simulink model "code_gen_man_bin"  (Simulink 7.5)
settings: Solver=FixedStepDiscrete  SolverMode=SingleTasking  StartTime=0.0  StopTime=10.0  FixedStep=0.01  RelTol=1e-3
InitFcn:
  | boat_constants
values from neighbouring files (symbols this model uses):
  figure8_waypoints = int32([ ... (first row only)    [boat_constants.m]
  InitialPoint = 0    [boat_constants.m]    (also in l2plus.m)
  IPStar = 0    [boat_constants.m]    (also in l2plus.m)
  ISA_g = 9.815    [boat_constants.m]
  MaxDwnPthStar = 1    [boat_constants.m]    (also in l2plus.m)
  OC2max = 49999    [boat_constants.m]    (also in simulation_constants.m)
  sampling_waypoints = int32([ ... (first row only)    [boat_constants.m]
  switchDistance = 4    [boat_constants.m]    (also in l2plus.m)
  T_step = 0.01    [boat_constants.m]    (also in common.m)
  tanIntercept = tan( 45*pi/180 )    [boat_constants.m]    (also in l2plus.m)
  test_waypoints = int32([ ... (first row only)    [boat_constants.m]
  TStar = single(4.5)    [boat_constants.m]    (also in l2plus.m = single(2))
  Turn2Track = 0    [boat_constants.m]    (also in l2plus.m)
  wheelbase = 3.27    [boat_constants.m]
undefined symbols (not defined in the file or in its folder): clearGpsData, clearSensorData, cpInitCommunications, DataEEInitAndClear, DataEEWrite, DiscIntNeverNeededParam, ecan1_buffered_transmit_matlab, ecan1_error_status_matlab, ecan1_init, GetAirData, getGpsData, getRevoData, getSensorData, GetThrottleData, GetWaterData, GetWindData, Init_onlyOnce, Init_Reset, initCalibrationRange, initGps, processNewCommData, processNewGpsData, processNewRevoData, setHilMode, u1, u2, uart1EnqueueStateData, uart2EnqueueActuatorData, y1
libraries: simulink x80, dsPICdrivers x50, uSimLib x4, simulink_need_slupdate x4
(part 3 of 6)

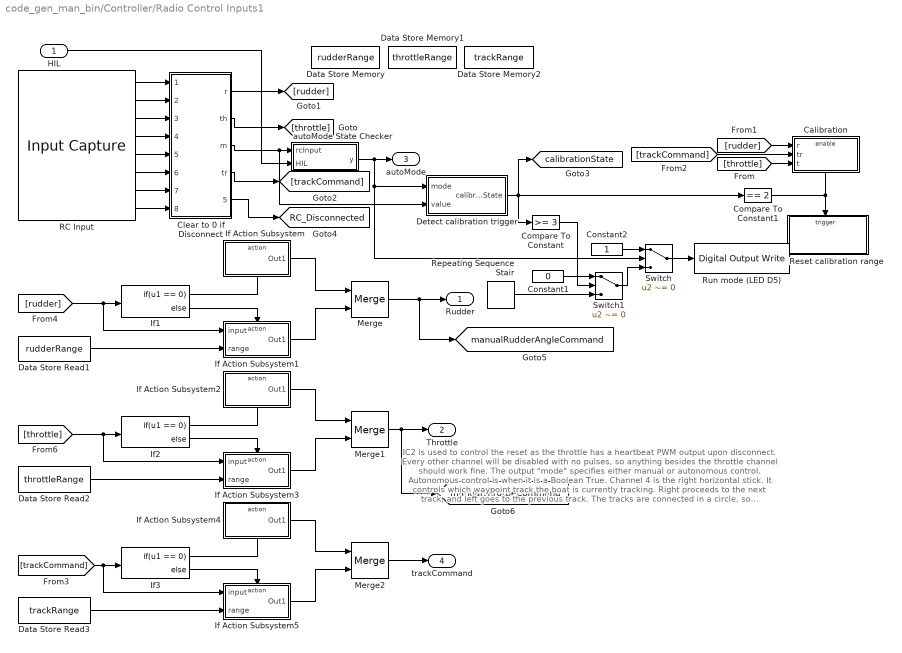
== system code_gen_man_bin/Controller/Radio Control Inputs1 ==
  note: IC2 is used to control the reset as the throttle has a heartbeat PWM output upon disconnect.
      | Every other channel will be disabled with no pulses, so anything besides the throttle channel
      | should work fine.
      |
      | The output "mode" specifies either manual or autonomous control. Autonomous control is when
      | it is a Boolean True.
      |
      | Channel 4 is the right horizontal stick. It controls which waypoint track the boat is currently tracking.
      | Right proceeds to the next track, and left goes to the previous track. The tracks are connected in a
      | circle, so next/prevTrack will eventually wrap around.
      |
      | All controls for the vehicle are controlled when AutoMode is True. When the vehicle is in
      | AutoMode, then its calibration features are engaged. Moving all control channels besides channel
      | 5 (which is reserved for switching AutoMode) will calibrate the controller to the proper values.
      |
      | As the vehicle enters reset automatically on startup, the proper way to calibrate is to startup the vehicle.
      | Move all the control sticks (excl channel 5 again) and then switch into RC mode. Even if the vessel stays
      | in reset mode, it will still be controllable via the RC transmitter.
      |
      | The output for rudder, throttle, and trackCommand are all in the range -1..1000. -1 means disconnected,
      | while 0 is a low RC signal and 1000 is a high. These ranges also have deadbands: 4% at the low-end or
      | 8% around the center. This helps to keep the actuator dead if the user desires it.
  HIL : Inport
  Calibration : Subsystem  TreatAsAtomicUnit=on
  Clear to 0 if Disconnect : Subsystem
  Compare To Constant : simulink/Logic and Bit Operations/Compare To Constant  SystemSampleTime=-1  relop=>=  const=3  LogicOutDataTypeMode=boolean
  Compare To Constant1 : simulink/Logic and Bit Operations/Compare To Constant  SystemSampleTime=-1  relop===  const=2  LogicOutDataTypeMode=boolean
  Constant1 : Constant  Value=0  OutDataTypeMode=boolean  OutDataType=fixdt(1, 16)  OutScaling=2^0  OutDataTypeStr=boolean
  Constant2 : Constant  OutDataTypeMode=boolean  OutDataType=fixdt(1, 16)  OutScaling=2^0  OutDataTypeStr=boolean
  Data Store Memory : DataStoreMemory  DataStoreName=rudderRange  ReadBeforeWriteMsg=warning  WriteAfterWriteMsg=warning  WriteAfterReadMsg=warning  InitialValue=[0 0]  DataType=int16  OutDataType=fixdt(1, 16)  OutScaling=2^0  OutDataTypeStr=int16
      settings: RTWStateStorageClass=ExportedGlobal
  Data Store Memory1 : DataStoreMemory  DataStoreName=throttleRange  ReadBeforeWriteMsg=warning  WriteAfterWriteMsg=warning  WriteAfterReadMsg=warning  InitialValue=[8000 8000]  DataType=int16  OutDataType=fixdt(1, 16)  OutScaling=2^0  OutDataTypeStr=int16
      settings: RTWStateStorageClass=ExportedGlobal
  Data Store Memory2 : DataStoreMemory  DataStoreName=trackRange  ReadBeforeWriteMsg=warning  WriteAfterWriteMsg=warning  WriteAfterReadMsg=warning  InitialValue=[8000 8000]  DataType=int16  OutDataType=fixdt(1, 16)  OutScaling=2^0  OutDataTypeStr=int16
      settings: RTWStateStorageClass=ExportedGlobal
  Data Store Read1 : DataStoreRead  DataStoreName=rudderRange  SampleTime=T_step
  Data Store Read2 : DataStoreRead  DataStoreName=throttleRange  SampleTime=T_step
  Data Store Read3 : DataStoreRead  DataStoreName=trackRange  SampleTime=T_step
  Detect calibration trigger : Subsystem
  If Action Subsystem : Subsystem  TreatAsAtomicUnit=on
  If Action Subsystem1 : Subsystem  TreatAsAtomicUnit=on
  If Action Subsystem2 : Subsystem  TreatAsAtomicUnit=on
  If Action Subsystem3 : Subsystem  TreatAsAtomicUnit=on
  If Action Subsystem4 : Subsystem  TreatAsAtomicUnit=on
  If Action Subsystem5 : Subsystem  TreatAsAtomicUnit=on
  If1 : If  IfExpression=u1 == 0
  If2 : If  IfExpression=u1 == 0
  If3 : If  IfExpression=u1 == 0
  Merge : Merge
  Merge1 : Merge
  Merge2 : Merge
  RC Input : dsPICdrivers/Peripheral I//O/Input Capture  Tag=dsPIC_PWM_IC  Priority=5  IntPriority=7  Channel=[2 3 4 8]  Channel_UP_Down_Periode="[1  1  1  1]"  MaxChannel="[0.0025      0.0025      0.0025      0.0025]"  SafeMarge="[1  1  1  1]"  MaxName=' IC2max , IC3max , IC4max , IC8max '  Precision="[13.6094      13.6094      13.6094      13.6094]"  Timer="[2  2  2  2]"  ChangeDetected="[2  2  2  2]"  ChangeDetectedPortRef=3  SampleTime=.01  Status=OK
  Repeating Sequence Stair : simulink/Sources/Repeating Sequence Stair  SystemSampleTime=-1  OutValues=[1 1 1 1 1 1 1 1 1 1 0 0 0 0 0 0 0 0 0 0]  tsamp=.01  OutMin=[]  OutMax=[]  OutDataTypeStr=fixdt('boolean')  OutputDataTypeScalingMode=Specify via dialog  OutDataType=fixdt('boolean')  ConRadixGroup=Best Precision: Vector-wise  OutScaling=[]
  Reset calibration range : Subsystem  TreatAsAtomicUnit=on
  Run mode (LED D5) : dsPICdrivers/Digital I//O/Digital Output Write  Tag=dsPIC_Digital_Output  Priority=5  PORT=A  Pin=[2]  Simultaneous=off  OrderingInOutPopup=None
  Switch : Switch  Criteria=u2 ~= 0  OutDataType=fixdt(1, 16)  OutScaling=2^0
  Switch1 : Switch  Criteria=u2 ~= 0  OutDataType=fixdt(1, 16)  OutScaling=2^0
  autoMode State Checker : Stateflow chart  TreatAsAtomicUnit=on
  Rudder : Outport
  Throttle : Outport  Port=2
  autoMode : Outport  Port=3
  trackCommand : Outport  Port=4
  tag scope: RC_Disconnected=global, calibrationState=global, manualRudderAngleCommand=global, manualThrottleCommand=global
  wires:
  Clear to 0 if Disconnect/3(m) -> Detect calibration trigger/2(value), autoMode State Checker/1(rcInput)
  Clear to 0 if Disconnect/1(r) -> [rudder]
  Clear to 0 if Disconnect/2(th) -> [throttle]
  Clear to 0 if Disconnect/4(tr) -> [trackCommand]
  [rudder] -> If Action Subsystem1/1(input), If1/1
  Data Store Read2/1 -> If Action Subsystem3/2(range)
  If1/1 -> If Action Subsystem/Action
  If1/2 -> If Action Subsystem1/Action
  If Action Subsystem1/1(Out1) -> Merge/2
  If Action Subsystem/1(Out1) -> Merge/1
  Data Store Read1/1 -> If Action Subsystem1/2(range)
  [throttle] -> If2/1, If Action Subsystem3/1(input)
  Merge1/1 -> Throttle/1, [manualThrottleCommand]
  If2/1 -> If Action Subsystem2/Action
  If2/2 -> If Action Subsystem3/Action
  If Action Subsystem3/1(Out1) -> Merge1/2
  If Action Subsystem2/1(Out1) -> Merge1/1
  [trackCommand] -> If3/1, If Action Subsystem5/1(input)
  Merge2/1 -> trackCommand/1
  If3/1 -> If Action Subsystem4/Action
  If3/2 -> If Action Subsystem5/Action
  If Action Subsystem5/1(Out1) -> Merge2/2
  If Action Subsystem4/1(Out1) -> Merge2/1
  Data Store Read3/1 -> If Action Subsystem5/2(range)
  autoMode State Checker/1(y) -> autoMode/1, Detect calibration trigger/1(mode), Switch/2
  Detect calibration trigger/1(calibrateState) -> Compare To Constant/1, Compare To Constant1/1, [calibrationState]
  [rudder] -> Calibration/1(r)
  [trackCommand] -> Calibration/2(tr)
  [throttle] -> Calibration/3(t)
  HIL/1 -> autoMode State Checker/2(HIL)
  Compare To Constant1/1 -> Reset calibration range/Trigger, Calibration/Enable
  Switch/1 -> Run mode (LED D5)/1
  Constant2/1 -> Switch/1
  Switch1/1 -> Switch/3
  Repeating Sequence Stair/1 -> Switch1/3
  Compare To Constant/1 -> Switch1/2
  Constant1/1 -> Switch1/1
  RC Input/1 -> Clear to 0 if Disconnect/1(rudder_up)
  RC Input/2 -> Clear to 0 if Disconnect/2(rudder_fall)
  RC Input/3 -> Clear to 0 if Disconnect/3(throttle_up)
  RC Input/4 -> Clear to 0 if Disconnect/4(throttle_fall)
  RC Input/5 -> Clear to 0 if Disconnect/5(mode_up)
  RC Input/6 -> Clear to 0 if Disconnect/6(mode_fall)
  RC Input/7 -> Clear to 0 if Disconnect/7(track_up)
  RC Input/8 -> Clear to 0 if Disconnect/8(track_fall)
  Clear to 0 if Disconnect/5(discon) -> [RC_Disconnected]
  Merge/1 -> Rudder/1, [manualRudderAngleCommand]

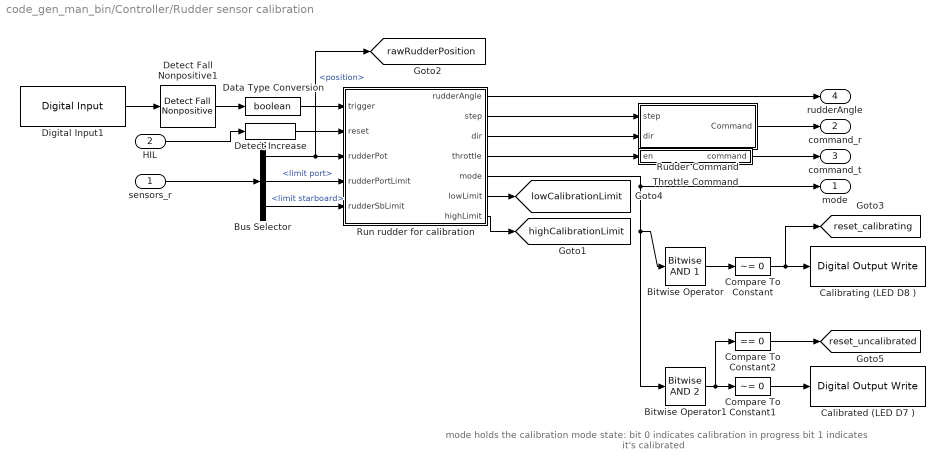
== system code_gen_man_bin/Controller/Rudder sensor calibration ==
  note: mode holds the calibration mode state:
      | bit 0 indicates calibration in progress
      | bit 1 indicates it's calibrated
  sensors_r : Inport
  HIL : Inport  Port=2
  Bitwise Operator : simulink/Logic and Bit Operations/Bitwise Operator  logicop=AND  UseBitMask=on  BitMask=1  BitMaskRealWorld=Stored Integer
  Bitwise Operator1 : simulink/Logic and Bit Operations/Bitwise Operator  logicop=AND  UseBitMask=on  BitMask=2  BitMaskRealWorld=Stored Integer
  Bus Selector : BusSelector  OutputSignals=position,limit port,limit starboard
  Calibrated (LED D7 ) : dsPICdrivers/Digital I//O/Digital Output Write  Tag=dsPIC_Digital_Output  Priority=5  PORT=A  Pin=[4]  Simultaneous=off  OrderingInOutPopup=None
  Calibrating (LED D8 ) : dsPICdrivers/Digital I//O/Digital Output Write  Tag=dsPIC_Digital_Output  Priority=5  PORT=A  Pin=[5]  Simultaneous=off  OrderingInOutPopup=None
  Compare To Constant : simulink/Logic and Bit Operations/Compare To Constant  SystemSampleTime=-1  relop=~=  const=0  LogicOutDataTypeMode=boolean
  Compare To Constant1 : simulink/Logic and Bit Operations/Compare To Constant  SystemSampleTime=-1  relop=~=  const=0  LogicOutDataTypeMode=boolean
  Compare To Constant2 : simulink/Logic and Bit Operations/Compare To Constant  SystemSampleTime=-1  relop===  const=0  LogicOutDataTypeMode=boolean
  Data Type Conversion : DataTypeConversion  OutDataTypeMode=boolean  OutDataType=fixdt(1, 16)  OutScaling=2^0  OutDataTypeStr=boolean
  Detect Increase : simulink/Logic and Bit Operations/Detect Increase  SystemSampleTime=-1  vinit=0.0
  Detect Fall Nonpositive1 : simulink/Logic and Bit Operations/Detect Fall Nonpositive  SystemSampleTime=-1  vinit=1
  Digital Input1 : dsPICdrivers/Digital I//O/Digital Input  Tag=dsPIC_Digital_Input  PORT=D  Pin=[7]  SampleTime=T_step  OrderingInOutPopup=None
  Rudder Command : Subsystem
  Run rudder for calibration : Stateflow chart  TreatAsAtomicUnit=on
  Throttle Command : Subsystem
  mode : Outport
  command_r : Outport  Port=2
  command_t : Outport  Port=3
  rudderAngle : Outport  Port=4
  tag scope: highCalibrationLimit=global, lowCalibrationLimit=global, rawRudderPosition=global, reset_calibrating=global, reset_uncalibrated=global
  wires:
  Digital Input1/1 -> Detect Fall Nonpositive1/1
  Detect Fall Nonpositive1/1 -> Data Type Conversion/1
  Data Type Conversion/1 -> Run rudder for calibration/1(trigger)
  Run rudder for calibration/2(step) -> Rudder Command/1(step)
  Run rudder for calibration/3(dir) -> Rudder Command/2(dir)
  Run rudder for calibration/4(throttle) -> Throttle Command/1(en)
  Throttle Command/1(command) -> command_t/1
  Rudder Command/1(Command) -> command_r/1
  Run rudder for calibration/5(mode) -> mode/1, Bitwise Operator/1, Bitwise Operator1/1
  Compare To Constant/1 -> Calibrating (LED D8 )/1, [reset_calibrating]
  Bitwise Operator/1 -> Compare To Constant/1
  Bitwise Operator1/1 -> Compare To Constant1/1, Compare To Constant2/1
  Compare To Constant1/1 -> Calibrated (LED D7 )/1
  Run rudder for calibration/1(rudderAngle) -> rudderAngle/1
  Run rudder for calibration/6(lowLimit) -> [lowCalibrationLimit]
  Run rudder for calibration/7(highLimit) -> [highCalibrationLimit]
  HIL/1 -> Detect Increase/1
  Detect Increase/1 -> Run rudder for calibration/2(reset)
  sensors_r/1 -> Bus Selector/1
  Bus Selector/2 -> Run rudder for calibration/4(rudderPortLimit)  "<limit port>"
  Bus Selector/3 -> Run rudder for calibration/5(rudderSbLimit)  "<limit starboard>"
  Bus Selector/1 -> Run rudder for calibration/3(rudderPot), [rawRudderPosition]  "<position>"
  Compare To Constant2/1 -> [reset_uncalibrated]

== system code_gen_man_bin/Controller/Sensor & GPS Reset ==
  note: When the processor gets reset be sure to
      | also reset the various structs that persist data:
      | specifically the GPS and Sensor structs.
  Trigger : TriggerPort  TriggerType=either
  Clear GPS struct [gps.c] : dsPICdrivers/OTHERS/C Function Call  Tag=dsPIC_dsPIC_CFunctionCall  FctUpdate=Output Function  fctName='clearGpsData'  INPUT_SIZE=1  INPUT1=--  INPUT2=--  INPUT3=--  OUTPUT_SIZE=1  OUTPUT1=--  SampleTime=-1  InputType=[ ]  OutputType=[ ]  FctDeclaration=extern void clearGpsData();  FctCall=clearGpsData();  OrderingInOutPopup=None  FctStart=None  FctStart_Name=Init_onlyOnce  FctStart_Declaration=inline extern void Init_onlyOnce();  FctStart_Call=Init_onlyOnce();  FctInit=None  FctInit_Name=Init_Reset  FctInit_Declaration=inline extern void Init_Reset();  FctInit_Call=Init_Reset();  PinDigitalInput=[]  PinDigitalOutput=[]  AnalogueInput=[]
  Clear sensor data struct [commProtocol.c] : dsPICdrivers/OTHERS/C Function Call  Tag=dsPIC_dsPIC_CFunctionCall  FctUpdate=Output Function  fctName='clearSensorData'  INPUT_SIZE=1  INPUT1=--  INPUT2=--  INPUT3=--  OUTPUT_SIZE=1  OUTPUT1=--  SampleTime=-1  InputType=[ ]  OutputType=[ ]  FctDeclaration=extern void clearSensorData();  FctCall=clearSensorData();  OrderingInOutPopup=None  FctStart=None  FctStart_Name=Init_onlyOnce  FctStart_Declaration=inline extern void Init_onlyOnce();  FctStart_Call=Init_onlyOnce();  FctInit=None  FctInit_Name=Init_Reset  FctInit_Declaration=inline extern void Init_Reset();  FctInit_Call=Init_Reset();  PinDigitalInput=[]  PinDigitalOutput=[]  AnalogueInput=[]

== system code_gen_man_bin/Controller/Split trackCommand to singular commands ==
  note: This block splits the trackCommand RC input into two control signals:
      | nextTrack - This is high to trigger switching to the next track of waypoints
      | resetTrack - This is high in order to reset the current track to the first one.
      | The transition between tracks can also only occur if the vehicle is in manual
      | control mode.
  autoMode : Inport
  trackCommand : Inport  Port=2
  Compare To Constant1 : simulink/Logic and Bit Operations/Compare To Constant  SystemSampleTime=-1  relop=>  const=800  LogicOutDataTypeMode=boolean
  Compare To Constant2 : simulink/Logic and Bit Operations/Compare To Constant  SystemSampleTime=-1  relop=<  const=200  LogicOutDataTypeMode=boolean
  Compare To Constant3 : simulink/Logic and Bit Operations/Compare To Constant  SystemSampleTime=-1  relop=~=  const=0  LogicOutDataTypeMode=boolean
  Countdown timer for trigger : Subsystem
  Countdown timer for trigger1 : Subsystem
  Logical Operator : Logic  Inputs=3  AllPortsSameDT=off  OutDataTypeMode=boolean  LogicDataType=fixdt(0, 8)  OutDataTypeStr=boolean
  Logical Operator1 : Logic  Inputs=3  AllPortsSameDT=off  OutDataTypeMode=boolean  LogicDataType=fixdt(0, 8)  OutDataTypeStr=boolean
  Logical Operator2 : Logic  Operator=NOT  Inputs=1  AllPortsSameDT=off  OutDataTypeMode=boolean  LogicDataType=fixdt(0, 8)  OutDataTypeStr=boolean
  nextTrack : Outport
  resetTrack : Outport  Port=2
  wires:
  Compare To Constant1/1 -> Logical Operator/1
  Compare To Constant2/1 -> Logical Operator1/1
  autoMode/1 -> Logical Operator2/1
  trackCommand/1 -> Compare To Constant1/1, Compare To Constant2/1, Compare To Constant3/1
  Logical Operator/1 -> Countdown timer for trigger/1(in)
  Countdown timer for trigger/1(trigger) -> nextTrack/1
  Logical Operator1/1 -> Countdown timer for trigger1/1(in)
  Countdown timer for trigger1/1(trigger) -> resetTrack/1
  Logical Operator2/1 -> Logical Operator/2, Logical Operator1/2
  Compare To Constant3/1 -> Logical Operator/3, Logical Operator1/3

== system code_gen_man_bin/Sensor Inputs/Atomic Subsystem ==
  HIL : Inport  OutDataType=fixdt(1, 16)  OutScaling=2^0
  GPS_g : Inport  Port=2  OutDataType=fixdt(1, 16)  OutScaling=2^0
  GPS_t : Inport  Port=3  OutDataType=fixdt(1, 16)  OutScaling=2^0
  Throttle_g : Inport  Port=4  OutDataType=fixdt(1, 16)  OutScaling=2^0
  Throttle_t : Inport  Port=5  OutDataType=fixdt(1, 16)  OutScaling=2^0
  Rudder_g : Inport  Port=6  OutDataType=fixdt(1, 16)  OutScaling=2^0
  Rudder_t : Inport  Port=7  OutDataType=fixdt(1, 16)  OutScaling=2^0
  Ballast_g : Inport  Port=8  OutDataType=fixdt(1, 16)  OutScaling=2^0
  Ballast_t : Inport  Port=9  OutDataType=fixdt(1, 16)  OutScaling=2^0
  HILSensorsMode : Inport  Port=10  OutDataType=fixdt(1, 16)  OutScaling=2^0
  Logical Operator : Logic  AllPortsSameDT=off  OutDataTypeMode=boolean  LogicDataType=fixdt(0, 8)  OutDataTypeStr=boolean
  Logical Operator1 : Logic  Operator=NOT  Inputs=1  AllPortsSameDT=off  OutDataTypeMode=boolean  LogicDataType=fixdt(0, 8)  OutDataTypeStr=boolean
  Switch{,1..3} (4 alike) : Switch  Criteria=u2 ~= 0  OutDataType=fixdt(1, 16)  OutScaling=2^0
  GPS : Outport  OutDataType=fixdt(1, 16)  OutScaling=2^0
  Throttle : Outport  Port=2  OutDataType=fixdt(1, 16)  OutScaling=2^0
  Rudder : Outport  Port=3  OutDataType=fixdt(1, 16)  OutScaling=2^0
  Ballast : Outport  Port=4  OutDataType=fixdt(1, 16)  OutScaling=2^0
  wires:
  HIL/1 -> Switch/2, Switch1/2, Switch3/2, Logical Operator/2
  GPS_g/1 -> Switch/1
  GPS_t/1 -> Switch/3
  Switch/1 -> GPS/1
  Throttle_g/1 -> Switch1/1
  Throttle_t/1 -> Switch1/3
  Switch1/1 -> Throttle/1
  Rudder_g/1 -> Switch2/1
  Rudder_t/1 -> Switch2/3
  Ballast_g/1 -> Switch3/1
  Ballast_t/1 -> Switch3/3
  Switch3/1 -> Ballast/1
  Switch2/1 -> Rudder/1
  HILSensorsMode/1 -> Logical Operator1/1
  Logical Operator1/1 -> Logical Operator/1
  Logical Operator/1 -> Switch2/2

== system code_gen_man_bin/Sensor Inputs/Ballast Sensors ==
  Bus Creator : BusCreator  Inputs=3
  Constant : Constant  Value=0  OutDataTypeMode=uint16  OutDataType=fixdt(1, 16)  OutScaling=2^0  OutDataTypeStr=uint16  SampleTime=T_step
  Constant1 : Constant  Value=0  OutDataTypeMode=boolean  OutDataType=fixdt(1, 16)  OutScaling=2^0  OutDataTypeStr=boolean  SampleTime=T_step
  Constant2 : Constant  Value=0  OutDataTypeMode=boolean  OutDataType=fixdt(1, 16)  OutScaling=2^0  OutDataTypeStr=boolean  SampleTime=T_step
  Out1 : Outport
  wires:
  Bus Creator/1 -> Out1/1
  Constant2/1 -> Bus Creator/3  "limit port"
  Constant1/1 -> Bus Creator/2  "limit starboard"
  Constant/1 -> Bus Creator/1  "position"

== system code_gen_man_bin/Sensor Inputs/Change UART Baudrate ==
  HIL : Inport
  Enable : EnablePort
  Data Type Conversion : DataTypeConversion  OutDataType=fixdt(1, 16)  OutScaling=2^0
  Reconfigure UART2 baud rate [commProtocol.c] : dsPICdrivers/OTHERS/C Function Call  Tag=dsPIC_dsPIC_CFunctionCall  FctUpdate=Output Function  fctName='setHilMode'  INPUT_SIZE=1  INPUT1=uint8  INPUT2=--  INPUT3=--  OUTPUT_SIZE=1  OUTPUT1=--  SampleTime=T_step  InputType=[ 2 ]  OutputType=[ ]  FctDeclaration=extern void setHilMode(uint8_T u1);  FctCall=setHilMode(%u1);  OrderingInOutPopup=None  FctStart=None  FctStart_Name=Init_onlyOnce  FctStart_Declaration=inline extern void Init_onlyOnce();  FctStart_Call=Init_onlyOnce();  FctInit=None  FctInit_Name=Init_Reset  FctInit_Declaration=inline extern void Init_Reset();  FctInit_Call=Init_Reset();  PinDigitalInput=[]  PinDigitalOutput=[]  AnalogueInput=[]
  wires:
  HIL/1 -> Data Type Conversion/1
  Data Type Conversion/1 -> Reconfigure UART2 baud rate [commProtocol.c]/1

== system code_gen_man_bin/Sensor Inputs/Estop detection ==
  note: If a status message hasn't been received for 2.1 seconds, a reset
      | signal is activated. The status messages for the ACS300 are not
      | sent when it is in reset, so this will catch when the estop is active.
      |
      | This also serves to check that the CAN hardware is working correctly,
      | which I have had trouble with in the past.
  Compare To Constant1 : simulink/Logic and Bit Operations/Compare To Constant  SystemSampleTime=-1  relop===  const=1  LogicOutDataTypeMode=boolean
  Constant1 : Constant  OutDataTypeMode=uint8  OutDataType=fixdt(1, 16)  OutScaling=2^0  OutDataTypeStr=uint8
  Discrete-Time Integrator : DiscreteIntegrator  IntegratorMethod=Accumulation: Forward Euler  gainval=1  ExternalReset=level  SampleTime=-1  OutDataType=fixdt(1, 16)  OutScaling=2^0  LimitOutput=on  UpperSaturationLimit=50  LowerSaturationLimit=0  ShowSaturationPort=on  ICPrevOutput=DiscIntNeverNeededParam  ICPrevScaledInput=DiscIntNeverNeededParam
  Retrieve throttle data from the ACS300 [ecanSensors.c] : dsPICdrivers/OTHERS/C Function Call  Tag=dsPIC_dsPIC_CFunctionCall  FctUpdate=Output Function  fctName=GetThrottleData  INPUT_SIZE=1  INPUT1=--  INPUT2=--  INPUT3=--  OUTPUT_SIZE=3  OUTPUT1=uint8  SampleTime=.01  InputType=[ ]  OutputType=[ 2 ]  FctDeclaration=extern void GetThrottleData(uint8_T* y1);  FctCall=GetThrottleData(*%y1);  OrderingInOutPopup=None  FctStart=None  FctStart_Name=Init_onlyOnce  FctStart_Declaration=inline extern void Init_onlyOnce();  FctStart_Call=Init_onlyOnce();  FctInit=None  FctInit_Name=Init_Reset  FctInit_Declaration=inline extern void Init_Reset();  FctInit_Call=Init_Reset();  PinDigitalInput=[]  PinDigitalOutput=[]  AnalogueInput=[]
  Terminator3 : Terminator
  Unpack throttle data : Stateflow chart  TreatAsAtomicUnit=on
  reset_estop : Outport
  tag scope: v_rpm=global
  wires:
  Retrieve throttle data from the ACS300 [ecanSensors.c]/1 -> Unpack throttle data/1(u)
  Unpack throttle data/1(throttle) -> [v_rpm]
  Constant1/1 -> Discrete-Time Integrator/1
  Unpack throttle data/2(newData) -> Discrete-Time Integrator/2
  Discrete-Time Integrator/2 -> Compare To Constant1/1
  Discrete-Time Integrator/1 -> Terminator3/1
  Compare To Constant1/1 -> reset_estop/1

== system code_gen_man_bin/Sensor Inputs/GPS ==
  Enable : EnablePort
  Bus Creator : BusCreator  Inputs=15
  Data Type Conversion : DataTypeConversion  OutDataTypeMode=boolean  OutDataType=fixdt(1, 16)  OutScaling=2^0  OutDataTypeStr=boolean  RndMeth=Simplest
  GPS Reception Status (LED D9) : dsPICdrivers/Digital I//O/Digital Output Write  Tag=dsPIC_Digital_Output  Priority=5  PORT=A  Pin=[6]  Simultaneous=off  OrderingInOutPopup=None
  Logical Operator4 : Logic  AllPortsSameDT=off  OutDataTypeMode=boolean  LogicDataType=fixdt(0, 8)  OutDataTypeStr=boolean
  Parse out new data since the last timestep [gps.c] : dsPICdrivers/OTHERS/C Function Call  Tag=dsPIC_dsPIC_CFunctionCall  FctUpdate=Output Function  fctName='processNewGpsData'  INPUT_SIZE=1  INPUT1=--  INPUT2=--  INPUT3=--  OUTPUT_SIZE=1  OUTPUT1=--  SampleTime=T_step  InputType=[ ]  OutputType=[ ]  FctDeclaration=extern void processNewGpsData();  FctCall=processNewGpsData();  OrderingInOutPopup=Output  FctStart=None  FctStart_Name=Init_onlyOnce  FctStart_Declaration=inline extern void Init_onlyOnce();  FctStart_Call=Init_onlyOnce();  FctInit=None  FctInit_Name=Init_Reset  FctInit_Declaration=inline extern void Init_Reset();  FctInit_Call=Init_Reset();  PinDigitalInput=[]  PinDigitalOutput=[]  AnalogueInput=[]
  Retrieve last GPS data [gps.c] : dsPICdrivers/OTHERS/C Function Call  Tag=dsPIC_dsPIC_CFunctionCall  FctUpdate=Output Function  fctName='getGpsData'  INPUT_SIZE=1  INPUT1=--  INPUT2=--  INPUT3=--  OUTPUT_SIZE=33  OUTPUT1=uint8  SampleTime=T_step  InputType=[ ]  OutputType=[ 2 ]  FctDeclaration=extern void getGpsData(uint8_T* y1);  FctCall=getGpsData(*%y1);  OrderingInOutPopup=Input  FctStart=None  FctStart_Name=Init_onlyOnce  FctStart_Declaration=inline extern void Init_onlyOnce();  FctStart_Call=Init_onlyOnce();  FctInit=None  FctInit_Name=Init_Reset  FctInit_Declaration=inline extern void Init_Reset();  FctInit_Call=Init_Reset();  PinDigitalInput=[]  PinDigitalOutput=[]  AnalogueInput=[]
  Unpack sensor data : Stateflow chart  TreatAsAtomicUnit=on
  GPS : Outport
  wires:
  Bus Creator/1 -> GPS/1
  Parse out new data since the last timestep [gps.c]/1 -> Retrieve last GPS data [gps.c]/1
  Data Type Conversion/1 -> Bus Creator/15, Logical Operator4/2  "newData"
  Unpack sensor data/15(newGpsData) -> Data Type Conversion/1
  Unpack sensor data/4(year) -> Bus Creator/4  "year"
  Unpack sensor data/5(month) -> Bus Creator/5  "month"
  Unpack sensor data/6(day) -> Bus Creator/6  "day"
  Unpack sensor data/7(hour) -> Bus Creator/7  "hour"
  Unpack sensor data/8(minute) -> Bus Creator/8  "minute"
  Unpack sensor data/9(second) -> Bus Creator/9  "second"
  Unpack sensor data/10(cog) -> Bus Creator/10  "cog"
  Unpack sensor data/11(sog) -> Bus Creator/11  "sog"
  Unpack sensor data/12(hdop) -> Bus Creator/12  "hdop"
  Unpack sensor data/13(fix) -> Bus Creator/13  "fix"
  Unpack sensor data/14(satellites) -> Bus Creator/14, Logical Operator4/1  "satellites"
  Retrieve last GPS data [gps.c]/1 -> Unpack sensor data/1(u)
  Unpack sensor data/1(latitude) -> Bus Creator/1  "latitude"
  Unpack sensor data/2(longitude) -> Bus Creator/2  "longitude"
  Unpack sensor data/3(altitude) -> Bus Creator/3  "altitude"
  Logical Operator4/1 -> GPS Reception Status (LED D9)/1

== system code_gen_man_bin/Sensor Inputs/Hold in reset on init ==
  note: This block outputs a 1 while it hasn't received 100 new and valid GPS fixes.
      | This counter gets reset on every transition to/from HIL mode.
  GPS : Inport
  HIL Button : Inport  Port=2
  Bus Selector : BusSelector  OutputSignals=newData,fix
  Compare To Zero : simulink/Logic and Bit Operations/Compare To Zero  SystemSampleTime=-1  relop===  LogicOutDataTypeMode=boolean
  Discrete-Time Integrator : DiscreteIntegrator  ExternalReset=either  SampleTime=-1  OutDataType=fixdt(1, 16)  OutScaling=2^0  LimitOutput=on  UpperSaturationLimit=1  LowerSaturationLimit=0  ICPrevOutput=DiscIntNeverNeededParam  ICPrevScaledInput=DiscIntNeverNeededParam
  Logical Operator : Logic  AllPortsSameDT=off  OutDataTypeMode=boolean  LogicDataType=fixdt(0, 8)  OutDataTypeStr=boolean
  Out1 : Outport
  wires:
  GPS/1 -> Bus Selector/1
  Compare To Zero/1 -> Out1/1
  Discrete-Time Integrator/1 -> Compare To Zero/1
  Bus Selector/1 -> Logical Operator/1  "<newData>"
  Bus Selector/2 -> Logical Operator/2  "<fix>"
  Logical Operator/1 -> Discrete-Time Integrator/1
  HIL Button/1 -> Discrete-Time Integrator/2

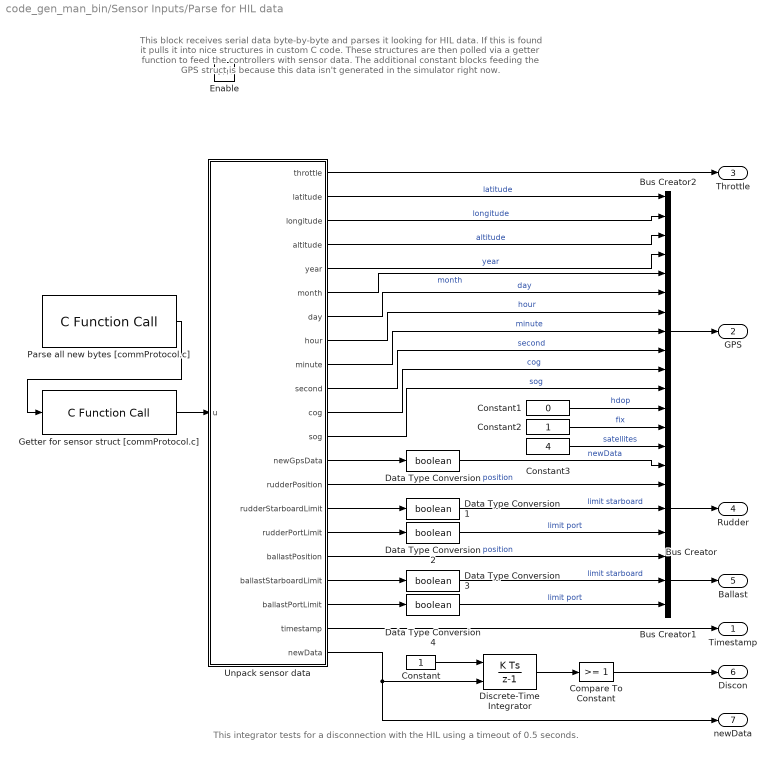
== system code_gen_man_bin/Sensor Inputs/Parse for HIL data ==
  note: This block receives serial data byte-by-byte and parses it looking for HIL data.
      | If this is found it pulls it into nice structures in custom C code. These structures
      | are then polled via a getter function to feed the controllers with sensor data.
      |
      | The additional constant blocks feeding the GPS struct is because this data isn't
      | generated in the simulator right now.
  note: This integrator tests for a disconnection with the HIL
      | using a timeout of 0.5 seconds.
  Enable : EnablePort
  Bus Creator : BusCreator  Inputs=3
  Bus Creator1 : BusCreator  Inputs=3
  Bus Creator2 : BusCreator  Inputs=15
  Compare To Constant : simulink/Logic and Bit Operations/Compare To Constant  SystemSampleTime=-1  relop=>=  const=1  LogicOutDataTypeMode=boolean
  Constant : Constant  OutDataTypeMode=uint8  OutDataType=fixdt(1, 16)  OutScaling=2^0  OutDataTypeStr=uint8
  Constant1 : Constant  Value=0  OutDataTypeMode=single  OutDataType=fixdt(1, 16)  OutScaling=2^0  OutDataTypeStr=single
  Constant2 : Constant  OutDataTypeMode=uint8  OutDataType=fixdt(1, 16)  OutScaling=2^0  OutDataTypeStr=uint8
  Constant3 : Constant  Value=4  OutDataTypeMode=uint8  OutDataType=fixdt(1, 16)  OutScaling=2^0  OutDataTypeStr=uint8
  Data Type Conversion{,1..4} (5 alike) : DataTypeConversion  OutDataTypeMode=boolean  OutDataType=fixdt(1, 16)  OutScaling=2^0  OutDataTypeStr=boolean
  Discrete-Time Integrator : DiscreteIntegrator  gainval=2  ExternalReset=level  SampleTime=T_step  OutDataType=fixdt(1, 16)  OutScaling=2^0  LimitOutput=on  UpperSaturationLimit=1  LowerSaturationLimit=0  ICPrevOutput=DiscIntNeverNeededParam  ICPrevScaledInput=DiscIntNeverNeededParam
  Getter for sensor struct [commProtocol.c] : dsPICdrivers/OTHERS/C Function Call  Tag=dsPIC_dsPIC_CFunctionCall  FctUpdate=Output Function  fctName='getSensorData'  INPUT_SIZE=1  INPUT1=--  INPUT2=--  INPUT3=--  OUTPUT_SIZE=40  OUTPUT1=uint8  SampleTime=.01  InputType=[ ]  OutputType=[ 2 ]  FctDeclaration=extern void getSensorData(uint8_T* y1);  FctCall=getSensorData(*%y1);  OrderingInOutPopup=Input  FctStart=None  FctStart_Name=Init_onlyOnce  FctStart_Declaration=inline extern void Init_onlyOnce();  FctStart_Call=Init_onlyOnce();  FctInit=None  FctInit_Name=Init_Reset  FctInit_Declaration=inline extern void Init_Reset();  FctInit_Call=Init_Reset();  PinDigitalInput=[]  PinDigitalOutput=[]  AnalogueInput=[]
  Parse all new bytes [commProtocol.c] : dsPICdrivers/OTHERS/C Function Call  Tag=dsPIC_dsPIC_CFunctionCall  FctUpdate=Output Function  fctName='processNewCommData'  INPUT_SIZE=1  INPUT1=--  INPUT2=--  INPUT3=--  OUTPUT_SIZE=1  OUTPUT1=--  SampleTime=.01  InputType=[ ]  OutputType=[ ]  FctDeclaration=extern void processNewCommData();  FctCall=processNewCommData();  OrderingInOutPopup=Output  FctStart=None  FctStart_Name=Init_onlyOnce  FctStart_Declaration=inline extern void Init_onlyOnce();  FctStart_Call=Init_onlyOnce();  FctInit=None  FctInit_Name=Init_Reset  FctInit_Declaration=inline extern void Init_Reset();  FctInit_Call=Init_Reset();  PinDigitalInput=[]  PinDigitalOutput=[]  AnalogueInput=[]
  Unpack sensor data : Stateflow chart  TreatAsAtomicUnit=on
  Timestamp : Outport
  GPS : Outport  Port=2
  Throttle : Outport  Port=3
  Rudder : Outport  Port=4
  Ballast : Outport  Port=5
  Discon : Outport  Port=6
  newData : Outport  Port=7
  wires:
  Unpack sensor data/1(throttle) -> Throttle/1
  Bus Creator/1 -> Rudder/1
  Bus Creator1/1 -> Ballast/1
  Bus Creator2/1 -> GPS/1
  Unpack sensor data/4(altitude) -> Bus Creator2/3  "altitude"
  Unpack sensor data/3(longitude) -> Bus Creator2/2  "longitude"
  Unpack sensor data/2(latitude) -> Bus Creator2/1  "latitude"
  Unpack sensor data/10(second) -> Bus Creator2/9  "second"
  Unpack sensor data/9(minute) -> Bus Creator2/8  "minute"
  Unpack sensor data/8(hour) -> Bus Creator2/7  "hour"
  Unpack sensor data/7(day) -> Bus Creator2/6  "day"
  Unpack sensor data/6(month) -> Bus Creator2/5  "month"
  Unpack sensor data/5(year) -> Bus Creator2/4  "year"
  Unpack sensor data/11(cog) -> Bus Creator2/10  "cog"
  Unpack sensor data/12(sog) -> Bus Creator2/11  "sog"
  Getter for sensor struct [commProtocol.c]/1 -> Unpack sensor data/1(u)
  Parse all new bytes [commProtocol.c]/1 -> Getter for sensor struct [commProtocol.c]/1
  Unpack sensor data/13(newGpsData) -> Data Type Conversion/1
  Unpack sensor data/14(rudderPosition) -> Bus Creator/1  "position"
  Unpack sensor data/15(rudderStarboardLimit) -> Data Type Conversion1/1
  Unpack sensor data/16(rudderPortLimit) -> Data Type Conversion2/1
  Unpack sensor data/17(ballastPosition) -> Bus Creator1/1  "position"
  Unpack sensor data/18(ballastStarboardLimit) -> Data Type Conversion3/1
  Unpack sensor data/19(ballastPortLimit) -> Data Type Conversion4/1
  Unpack sensor data/20(timestamp) -> Timestamp/1
  Constant/1 -> Discrete-Time Integrator/1
  Discrete-Time Integrator/1 -> Compare To Constant/1
  Unpack sensor data/21(newData) -> Discrete-Time Integrator/2, newData/1
  Compare To Constant/1 -> Discon/1
  Constant1/1 -> Bus Creator2/12  "hdop"
  Constant2/1 -> Bus Creator2/13  "fix"
  Constant3/1 -> Bus Creator2/14  "satellites"
  Data Type Conversion/1 -> Bus Creator2/15  "newData"
  Data Type Conversion1/1 -> Bus Creator/2  "limit starboard"
  Data Type Conversion2/1 -> Bus Creator/3  "limit port"
  Data Type Conversion3/1 -> Bus Creator1/2  "limit starboard"
  Data Type Conversion4/1 -> Bus Creator1/3  "limit port"

== system code_gen_man_bin/Sensor Inputs/RevoGS ==
  Enable : EnablePort
  Bus Creator : BusCreator  Inputs=9
  Parse out new data since the last timestep [revo.c] : dsPICdrivers/OTHERS/C Function Call  Tag=dsPIC_dsPIC_CFunctionCall  FctUpdate=Output Function  fctName=processNewRevoData  INPUT_SIZE=1  INPUT1=--  INPUT2=--  INPUT3=--  OUTPUT_SIZE=1  OUTPUT1=--  SampleTime=0.01  InputType=[ ]  OutputType=[ ]  FctDeclaration=extern void processNewRevoData();  FctCall=processNewRevoData();  OrderingInOutPopup=Output  FctStart=None  FctStart_Name=Init_onlyOnce  FctStart_Declaration=inline extern void Init_onlyOnce();  FctStart_Call=Init_onlyOnce();  FctInit=None  FctInit_Name=Init_Reset  FctInit_Declaration=inline extern void Init_Reset();  FctInit_Call=Init_Reset();  PinDigitalInput=[]  PinDigitalOutput=[]  AnalogueInput=[]
  Retrieve latest Revo data [revo.c] : dsPICdrivers/OTHERS/C Function Call  Tag=dsPIC_dsPIC_CFunctionCall  FctUpdate=Output Function  fctName=getRevoData  INPUT_SIZE=1  INPUT1=--  INPUT2=--  INPUT3=--  OUTPUT_SIZE=22  OUTPUT1=uint8  SampleTime=0.01  InputType=[ ]  OutputType=[ 2 ]  FctDeclaration=extern void getRevoData(uint8_T* y1);  FctCall=getRevoData(*%y1);  OrderingInOutPopup=Input  FctStart=None  FctStart_Name=Init_onlyOnce  FctStart_Declaration=inline extern void Init_onlyOnce();  FctStart_Call=Init_onlyOnce();  FctInit=None  FctInit_Name=Init_Reset  FctInit_Declaration=inline extern void Init_Reset();  FctInit_Call=Init_Reset();  PinDigitalInput=[]  PinDigitalOutput=[]  AnalogueInput=[]
  Unpack sensor data : Stateflow chart  TreatAsAtomicUnit=on
  RevoGS : Outport
  wires:
  Bus Creator/1 -> RevoGS/1
  Parse out new data since the last timestep [revo.c]/1 -> Retrieve latest Revo data [revo.c]/1
  Unpack sensor data/4(pitchStatus) -> Bus Creator/4  "pitchStatus"
  Unpack sensor data/5(roll) -> Bus Creator/5  "roll"
  Unpack sensor data/6(rollStatus) -> Bus Creator/6  "rollStatus"
  Unpack sensor data/7(dip) -> Bus Creator/7  "dip"
  Unpack sensor data/8(magneticMagnitude) -> Bus Creator/8  "magneticMagnitude"
  Unpack sensor data/9(newData) -> Bus Creator/9  "newData"
  Retrieve latest Revo data [revo.c]/1 -> Unpack sensor data/1(u)
  Unpack sensor data/1(heading) -> Bus Creator/1  "heading"
  Unpack sensor data/2(magStatus) -> Bus Creator/2  "magStatus"
  Unpack sensor data/3(pitch) -> Bus Creator/3  "pitch"

== system code_gen_man_bin/Sensor Inputs/Rudder Sensors ==
  note: The rudder has two main sensors: hall effect and a potentiometer. The
      | potentiometer returns a voltage value through the onboard ADC indicating
      | rudder position exactly. The three Hall effect sensors are used as limit switches
      | indicating port and starboard limits as well as center, though this sensor isn't
      | being used currently.
      |
      | It expects a range of 1.12-2.11V for the rudder position potentiometer with
      | 2.11V being hard to port. The potentiometer was powered at 3.3V for these
      | measurements.
  ADC in : Inport  OutDataType=fixdt(1, 16)  OutScaling=2^0
  Bus Creator : BusCreator  Inputs=3
  Logical Operator : Logic  Operator=NOT  Inputs=1  AllPortsSameDT=off  OutDataTypeMode=boolean  LogicDataType=fixdt(0, 8)  OutDataTypeStr=boolean
  Logical Operator1 : Logic  Operator=NOT  Inputs=1  AllPortsSameDT=off  OutDataTypeMode=boolean  LogicDataType=fixdt(0, 8)  OutDataTypeStr=boolean
  Port Hall : dsPICdrivers/Digital I//O/Digital Input  Tag=dsPIC_Digital_Input  PORT=C  Pin=[2]  SampleTime=.01  OrderingInOutPopup=None
  Starboard Hall : dsPICdrivers/Digital I//O/Digital Input  Tag=dsPIC_Digital_Input  PORT=G  Pin=[3]  SampleTime=.01  OrderingInOutPopup=None
  Weighted Moving Average : simulink_need_slupdate/Weighted Moving Average  mgainval=[.25 .25 .25 .25]  vinit=0.0  samptime=-1  OutDataTypeStr=Inherit: Inherit via back propagation  OutDataType=sfix(16)  OutScaling=2^-10  DoSatur=off  GainDataType=uint(16)  MatRadixGroup=Best Precision: Matrix-wise  GainScaling=2^-10
  Out1 : Outport
  wires:
  ADC in/1 -> Weighted Moving Average/1
  Starboard Hall/1 -> Logical Operator1/1
  Port Hall/1 -> Logical Operator/1
  Bus Creator/1 -> Out1/1
  Logical Operator/1 -> Bus Creator/3  "limit port"
  Logical Operator1/1 -> Bus Creator/2  "limit starboard"
  Weighted Moving Average/1 -> Bus Creator/1  "position"

== system code_gen_man_bin/Sensor Inputs/Throttle Sensors ==
  note: Throttle output is currently being ignored. The motor driver board
      | should report current velocity along with other status information
      | on a regular basis and that could be parsed for this information. As
      | of right now it's been deemed non-critical and therefore ignored.
  Constant : Constant  Value=0  OutDataTypeMode=int16  OutDataType=fixdt(1, 16)  OutScaling=2^0  OutDataTypeStr=int16  SampleTime=.01
  Out1 : Outport
  wires:
  Constant/1 -> Out1/1

== system code_gen_man_bin/Transmit actuator data/Package and Transmit Sensor Struct ==
  command_r : Inport
  command_b : Inport  Port=2
  command_t : Inport  Port=3
  timstamp : Inport  Port=4
  rudderAngle : Inport  Port=5
  sensorOverride : Inport  Port=6
  Enable : EnablePort
  Add actuator commands to transmission FIFO [commProtocol.c] : dsPICdrivers/OTHERS/C Function Call  Tag=dsPIC_dsPIC_CFunctionCall  FctUpdate=Output Function  fctName='uart2EnqueueActuatorData'  INPUT_SIZE=34  INPUT1=uint8  INPUT2=--  INPUT3=--  OUTPUT_SIZE=1  OUTPUT1=--  SampleTime=-1  InputType=[ 2 ]  OutputType=[ ]  FctDeclaration=extern void uart2EnqueueActuatorData(uint8_T* u1);  FctCall=uart2EnqueueActuatorData(*%u1);  OrderingInOutPopup=None  FctStart=None  FctStart_Name=Init_onlyOnce  FctStart_Declaration=inline extern void Init_onlyOnce();  FctStart_Call=Init_onlyOnce();  FctInit=None  FctInit_Name=Init_Reset  FctInit_Declaration=inline extern void Init_Reset();  FctInit_Call=Init_Reset();  PinDigitalInput=[]  PinDigitalOutput=[]  AnalogueInput=[]
  Build HIL sentence : Subsystem
  Bus Selector : BusSelector  OutputSignals=enable,direction,up,period
  Bus Selector1 : BusSelector  OutputSignals=identifier,data,size,trigger
  Bus Selector2 : BusSelector  OutputSignals=enable,direction
  Pack : Stateflow chart  TreatAsAtomicUnit=on
  wires:
  Bus Selector/2 -> Pack/2(r_dir)  "<direction>"
  Bus Selector/1 -> Pack/1(r_en)  "<enable>"
  Bus Selector1/4 -> Pack/10(t_trig)  "<trigger>"
  Bus Selector1/1 -> Pack/7(t_id)  "<identifier>"
  Bus Selector/3 -> Pack/3(r_up)  "<up>"
  Bus Selector2/1 -> Pack/5(b_en)  "<enable>"
  Bus Selector2/2 -> Pack/6(b_dir)  "<direction>"
  Bus Selector/4 -> Pack/4(r_per)  "<period>"
  Bus Selector1/2 -> Pack/8(t_data)  "<data>"
  Bus Selector1/3 -> Pack/9(t_size)  "<size>"
  command_r/1 -> Bus Selector/1
  command_b/1 -> Bus Selector2/1
  command_t/1 -> Bus Selector1/1
  timstamp/1 -> Pack/11(time)
  Build HIL sentence/1(sent) -> Add actuator commands to transmission FIFO [commProtocol.c]/1
  Pack/1(y) -> Build HIL sentence/1(data)
  rudderAngle/1 -> Pack/12(rudderAngle)
  sensorOverride/1 -> Pack/13(sensorOverride)

== system code_gen_man_bin/Transmit state data via UART1/Build HIL sentence ==
  data : Inport
  Bitwise Operator : simulink/Logic and Bit Operations/Bitwise Operator  logicop=XOR  UseBitMask=off  BitMask=bin2dec('11011001')  BitMaskRealWorld=Stored Integer
  Constant : Constant  Value=37  OutDataTypeMode=uint8  OutDataType=fixdt(1, 16)  OutScaling=2^0  OutDataTypeStr=uint8
  Constant1 : Constant  Value=38  OutDataTypeMode=uint8  OutDataType=fixdt(1, 16)  OutScaling=2^0  OutDataTypeStr=uint8
  Constant2 : Constant  Value=94  OutDataTypeMode=uint8  OutDataType=fixdt(1, 16)  OutScaling=2^0  OutDataTypeStr=uint8
  Constant3 : Constant  Value=38  OutDataTypeMode=uint8  OutDataType=fixdt(1, 16)  OutScaling=2^0  OutDataTypeStr=uint8
  Constant4 : Constant  Value=3  OutDataTypeMode=uint8  OutDataType=fixdt(1, 16)  OutScaling=2^0  OutDataTypeStr=uint8
  Mux2 : Mux  Inputs=3
  Pack : Stateflow chart  TreatAsAtomicUnit=on
  Probe : Probe  ProbeSampleTime=off  ProbeComplexSignal=off  ProbeWidthDataType=uint8
  sent : Outport
  wires:
  data/1 -> Probe/1, Mux2/3
  Constant/1 -> Pack/1(a)
  Constant1/1 -> Pack/2(b)
  Pack/1(y) -> sent/1
  Mux2/1 -> Bitwise Operator/1, Pack/3(c)
  Probe/1 -> Mux2/2
  Constant2/1 -> Pack/4(d)
  Constant3/1 -> Pack/5(e)
  Bitwise Operator/1 -> Pack/6(f)
  Constant4/1 -> Mux2/1

== system code_gen_man_bin/Actuator Outputs/To Drive Motor/C-function Call ==
  parameters : Inport  OutDataType=sfix(16)  OutScaling=2^0
  Enable : EnablePort
  ECAN1 Transmit [ecanFunctions.c] : dsPICdrivers/OTHERS/C Function Call  Tag=dsPIC_dsPIC_CFunctionCall  FctUpdate=Output Function  fctName='ecan1_buffered_transmit_matlab'  INPUT_SIZE=8  INPUT1=uint16  INPUT2=--  INPUT3=--  OUTPUT_SIZE=1  OUTPUT1=--  SampleTime=c_func_sample_time  InputType=[ 4 ]  OutputType=[ ]  FctDeclaration=extern void ecan1_buffered_transmit_matlab(uint16_T* u1);  FctCall=ecan1_buffered_transmit_matlab(*%u1);  OrderingInOutPopup=None  FctStart=None  FctStart_Name=Init_onlyOnce  FctStart_Declaration=inline extern void Init_onlyOnce();  FctStart_Call=Init_onlyOnce();  FctInit=None  FctInit_Name=Init_Reset  FctInit_Declaration=inline extern void Init_Reset();  FctInit_Call=Init_Reset();  PinDigitalInput=[]  PinDigitalOutput=[]  AnalogueInput=[]
  wires:
  parameters/1 -> ECAN1 Transmit [ecanFunctions.c]/1

== system code_gen_man_bin/Actuator Outputs/To Drive Motor/uint8 combiner1 ==
  high-order : Inport  OutDataType=sfix(16)  OutScaling=2^0
  low-order : Inport  Port=2  OutDataType=sfix(16)  OutScaling=2^0
  Bitwise Operator : simulink/Logic and Bit Operations/Bitwise Operator  logicop=OR  UseBitMask=off  NumInputPorts=2  BitMask=bin2dec('11011001')  BitMaskRealWorld=Stored Integer
  Data Type Conversion : DataTypeConversion  OutDataTypeMode=uint16  OutDataType=sfix(16)  OutScaling=2^0  OutDataTypeStr=uint16
  Data Type Conversion1 : DataTypeConversion  OutDataTypeMode=uint16  OutDataType=sfix(16)  OutScaling=2^0  OutDataTypeStr=uint16
  Shift Arithmetic : simulink/Logic and Bit Operations/Shift Arithmetic  SystemSampleTime=-1  nBitShiftRight=-8  nBinPtShiftRight=0
  combined : Outport  OutDataType=sfix(16)  OutScaling=2^0
  wires:
  low-order/1 -> Data Type Conversion/1
  Bitwise Operator/1 -> combined/1
  high-order/1 -> Data Type Conversion1/1
  Shift Arithmetic/1 -> Bitwise Operator/2
  Data Type Conversion/1 -> Shift Arithmetic/1
  Data Type Conversion1/1 -> Bitwise Operator/1

== system code_gen_man_bin/Actuator Outputs/To Drive Motor/uint8 combiner2 ==
  high-order : Inport  OutDataType=sfix(16)  OutScaling=2^0
  low-order : Inport  Port=2  OutDataType=sfix(16)  OutScaling=2^0
  Bitwise Operator : simulink/Logic and Bit Operations/Bitwise Operator  logicop=OR  UseBitMask=off  NumInputPorts=2  BitMask=bin2dec('11011001')  BitMaskRealWorld=Stored Integer
  Data Type Conversion : DataTypeConversion  OutDataTypeMode=uint16  OutDataType=sfix(16)  OutScaling=2^0  OutDataTypeStr=uint16
  Data Type Conversion1 : DataTypeConversion  OutDataTypeMode=uint16  OutDataType=sfix(16)  OutScaling=2^0  OutDataTypeStr=uint16
  Shift Arithmetic : simulink/Logic and Bit Operations/Shift Arithmetic  SystemSampleTime=-1  nBitShiftRight=-8  nBinPtShiftRight=0
  combined : Outport  OutDataType=sfix(16)  OutScaling=2^0
  wires:
  Data Type Conversion1/1 -> Bitwise Operator/1
  Data Type Conversion/1 -> Shift Arithmetic/1
  Shift Arithmetic/1 -> Bitwise Operator/2
  high-order/1 -> Data Type Conversion1/1
  Bitwise Operator/1 -> combined/1
  low-order/1 -> Data Type Conversion/1

== system code_gen_man_bin/Controller/Auto/Manual Switch/If Action Subsystem ==
  r_i : Inport  OutDataType=fixdt(1, 16)  OutScaling=2^0
  t_i : Inport  Port=2  OutDataType=fixdt(1, 16)  OutScaling=2^0
  Action Port : ActionPort  ActionType=else
  Signal Conversion : SignalConversion  ConversionOutput=Bus copy
  Signal Conversion1 : SignalConversion  ConversionOutput=Bus copy
  r_o : Outport  OutDataType=fixdt(1, 16)  OutScaling=2^0
  t_o : Outport  Port=2  OutDataType=fixdt(1, 16)  OutScaling=2^0
  wires:
  r_i/1 -> Signal Conversion/1
  t_i/1 -> Signal Conversion1/1
  Signal Conversion/1 -> r_o/1
  Signal Conversion1/1 -> t_o/1

== system code_gen_man_bin/Controller/Auto/Manual Switch/If Action Subsystem1 ==
  r_i : Inport  OutDataType=fixdt(1, 16)  OutScaling=2^0
  t_i : Inport  Port=2  OutDataType=fixdt(1, 16)  OutScaling=2^0
  Action Port : ActionPort  ActionType=then
  Signal Conversion : SignalConversion  ConversionOutput=Bus copy
  Signal Conversion1 : SignalConversion  ConversionOutput=Bus copy
  r_o : Outport  OutDataType=fixdt(1, 16)  OutScaling=2^0
  t_o : Outport  Port=2  OutDataType=fixdt(1, 16)  OutScaling=2^0
  wires:
  r_i/1 -> Signal Conversion1/1
  t_i/1 -> Signal Conversion/1
  Signal Conversion/1 -> t_o/1
  Signal Conversion1/1 -> r_o/1

== system code_gen_man_bin/Controller/Auto/Manual Switch/If Action Subsystem2 ==
  r_i : Inport  OutDataType=fixdt(1, 16)  OutScaling=2^0
  t_i : Inport  Port=2  OutDataType=fixdt(1, 16)  OutScaling=2^0
  Action Port : ActionPort  ActionType=else
  Signal Conversion : SignalConversion  ConversionOutput=Bus copy
  Signal Conversion1 : SignalConversion  ConversionOutput=Bus copy
  r_o : Outport  OutDataType=fixdt(1, 16)  OutScaling=2^0
  t_o : Outport  Port=2  OutDataType=fixdt(1, 16)  OutScaling=2^0
  wires:
  r_i/1 -> Signal Conversion/1
  t_i/1 -> Signal Conversion1/1
  Signal Conversion/1 -> r_o/1
  Signal Conversion1/1 -> t_o/1

== system code_gen_man_bin/Controller/Auto/Manual Switch/If Action Subsystem3 ==
  r_i : Inport  OutDataType=fixdt(1, 16)  OutScaling=2^0
  t_i : Inport  Port=2  OutDataType=fixdt(1, 16)  OutScaling=2^0
  Action Port : ActionPort  ActionType=then
  Signal Conversion : SignalConversion  ConversionOutput=Bus copy
  Signal Conversion1 : SignalConversion  ConversionOutput=Bus copy
  r_o : Outport  OutDataType=fixdt(1, 16)  OutScaling=2^0
  t_o : Outport  Port=2  OutDataType=fixdt(1, 16)  OutScaling=2^0
  wires:
  r_i/1 -> Signal Conversion1/1
  t_i/1 -> Signal Conversion/1
  Signal Conversion/1 -> t_o/1
  Signal Conversion1/1 -> r_o/1

== system code_gen_man_bin/Controller/Autonomous Controller/Ballast Command ==
  Bus Creator : BusCreator  Inputs=2
  Constant : Constant  Value=0  OutDataTypeMode=boolean  OutDataType=fixdt(1, 16)  OutScaling=2^0  OutDataTypeStr=boolean
  Constant1 : Constant  Value=0  OutDataTypeMode=boolean  OutDataType=fixdt(1, 16)  OutScaling=2^0  OutDataTypeStr=boolean
  c_ballast : Outport
  wires:
  Bus Creator/1 -> c_ballast/1
  Constant/1 -> Bus Creator/1  "enable"
  Constant1/1 -> Bus Creator/2  "direction"
